simulink model "net_model_2_nodes"  (R2024a)
settings: Solver=VariableStepAuto  StartTime=0.0  StopTime=100  RelTol=1e-3
values from neighbouring files (symbols this model uses):
  A = [A11, A12 ... (first row only)    [main.m]
  B = blkdiag(B, B)    [main.m]
  C = blkdiag(C, C)    [main.m]
  L = [0, 1 ... (first row only)    [main.m]
  node_1_0 = [0; 0]    [main.m]
  node_2_0 = [0; 0]    [main.m]
settings Model: Creator=antoniostavarache  LastModifiedBy=antoniostavarache

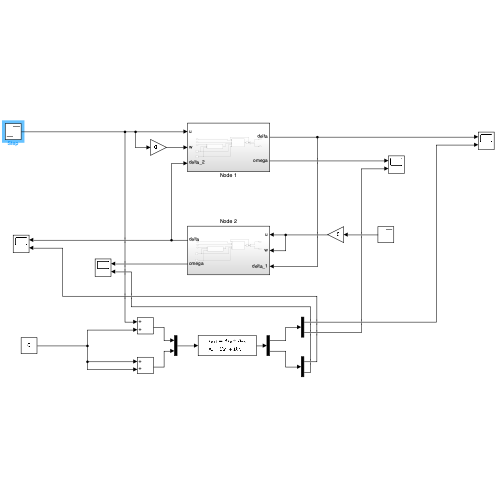
[thumbnail: Simulink's stored preview of the top-level diagram]
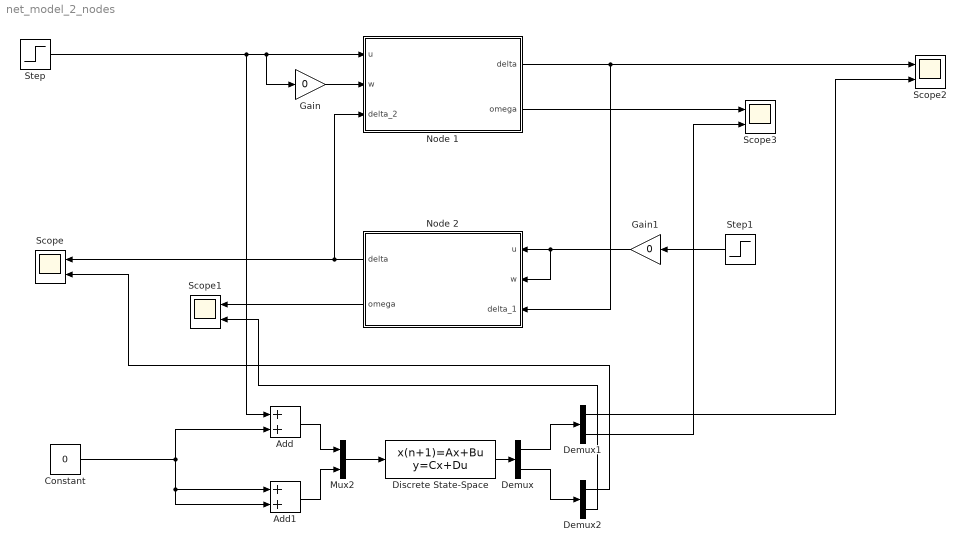
== system net_model_2_nodes ==
  Add : Sum
  Add1 : Sum
  Constant : Constant  Value=0
  Demux : Demux  Outputs=2
  Demux1 : Demux  Outputs=2
  Demux2 : Demux  Outputs=2
  Discrete State-Space : DiscreteStateSpace  A=A  B=B  C=C  D=zeros(4, 2)
  Gain : Gain  Gain=0
  Gain1 : Gain  Gain=0
  Mux2 : Mux  Inputs=2
  Node 1 : Subsystem
  Node 2 : Subsystem
  Scope{,1..3} (4 alike) : Scope  NumInputPorts=2
  Step : Step  SampleTime=0
  Step1 : Step  SampleTime=0
  wires:
  Node 1/1(delta) -> Scope2/1, Node 2/3(delta_1)
  Node 2/1(delta) -> Node 1/3(delta_2), Scope/1
  Node 2/2(omega) -> Scope1/1
  Node 1/2(omega) -> Scope3/1
  Step/1 -> Add/1, Node 1/1(u), Gain/1
  Gain/1 -> Node 1/2(w)
  Step1/1 -> Gain1/1
  Gain1/1 -> Node 2/2(w), Node 2/1(u)
  Constant/1 -> Add1/2, Add1/1, Add/2
  Add/1 -> Mux2/1
  Add1/1 -> Mux2/2
  Demux/1 -> Demux1/1
  Demux/2 -> Demux2/1
  Demux1/1 -> Scope2/2
  Demux1/2 -> Scope3/2
  Demux2/1 -> Scope/2
  Demux2/2 -> Scope1/2
  Mux2/1 -> Discrete State-Space/1
  Discrete State-Space/1 -> Demux/1

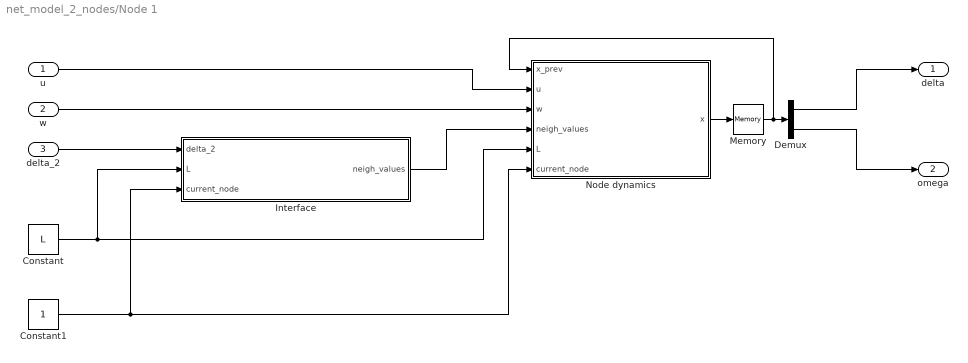
== system net_model_2_nodes/Node 1 ==
  u : Inport
  w : Inport  Port=2
  delta_2 : Inport  Port=3
  Constant : Constant  Value=L
  Constant1 : Constant
  Demux : Demux  Outputs=2
  Interface : MATLAB Function  TreatAsAtomicUnit=on
  Memory : Memory  InitialCondition=node_1_0
  Node dynamics : MATLAB Function  TreatAsAtomicUnit=on
  delta : Outport
  omega : Outport  Port=2
  wires:
  Node dynamics/1(x) -> Memory/1
  Interface/1(neigh_values) -> Node dynamics/4(neigh_values)
  Constant/1 -> Node dynamics/5(L), Interface/2(L)
  Constant1/1 -> Node dynamics/6(current_node), Interface/3(current_node)
  u/1 -> Node dynamics/2(u)
  w/1 -> Node dynamics/3(w)
  Demux/1 -> delta/1
  Demux/2 -> omega/1
  delta_2/1 -> Interface/1(delta_2)
  Memory/1 -> Node dynamics/1(x_prev), Demux/1

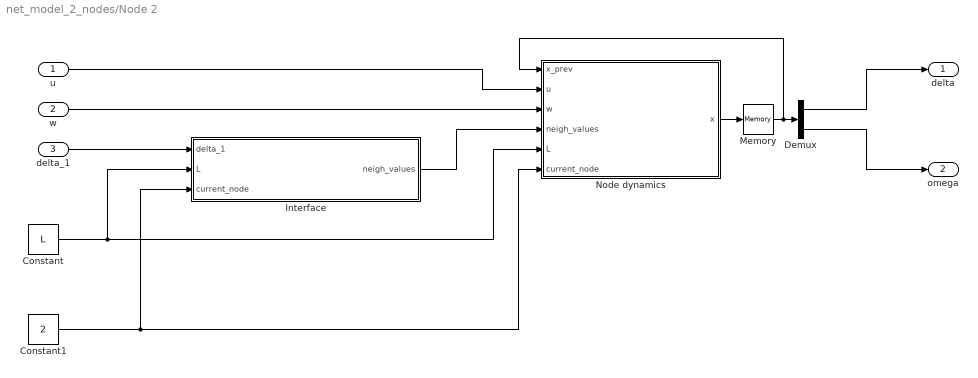
== system net_model_2_nodes/Node 2 ==
  u : Inport
  w : Inport  Port=2
  delta_1 : Inport  Port=3
  Constant : Constant  Value=L
  Constant1 : Constant  Value=2
  Demux : Demux  Outputs=2
  Interface : MATLAB Function  TreatAsAtomicUnit=on
  Memory : Memory  InitialCondition=node_2_0
  Node dynamics : MATLAB Function  TreatAsAtomicUnit=on
  delta : Outport
  omega : Outport  Port=2
  wires:
  Node dynamics/1(x) -> Memory/1
  Interface/1(neigh_values) -> Node dynamics/4(neigh_values)
  Constant/1 -> Node dynamics/5(L), Interface/2(L)
  Constant1/1 -> Node dynamics/6(current_node), Interface/3(current_node)
  u/1 -> Node dynamics/2(u)
  w/1 -> Node dynamics/3(w)
  Demux/1 -> delta/1
  Demux/2 -> omega/1
  delta_1/1 -> Interface/1(delta_1)
  Memory/1 -> Node dynamics/1(x_prev), Demux/1

== matlab function net_model_2_nodes/Node 1/Interface ==
  data: delta_2 input; neigh_values output; L input; current_node input
function neigh_values = fcn(delta_2, L, current_node)
    
    % curr_node = 1;

    % l_mat = [0 0.6511 0.7915 0 0.7513;
    %     0.6511 0 0 0.8433 0.6318;
    %     0.7915 0 0 0.8259 0.8620;
    %     0 0.8433 0.8259 0 0.8367;
    %     0.7513 0.6318 0.8620 0.8367 0];

    l_mat = [0 0.6511;
        0.6511 0];

    neigh_values = L(current_node, 2) * l_mat(current_node, 2) * delta_2;

end

== matlab function net_model_2_nodes/Node 1/Node dynamics ==
  data: x_prev input; u input; x output; w input; neigh_values input; L input; current_node input
function x = fcn(x_prev, u, w, neigh_values, L, current_node)
    
    % current_node = 1;

%%

    hi = [0.3244
        1.5886];

    di = [0.5650;
        0.7844];
    
    l_mat = [0 0.6511;
        0.6511 0];

    dt = 0.2;
%%

    a21 = -hi(current_node) * dt * L(current_node, :) * l_mat(current_node, :)';
    a22 = 1 - hi(current_node) * di(current_node) * dt;

    A = [1, dt;
        a21, a22];

    x = A * x_prev + [0 1]' * (u + w + hi(current_node) * dt * neigh_values);
    
end

== matlab function net_model_2_nodes/Node 2/Interface ==
  data: delta_1 input; neigh_values output; L input; current_node input
function neigh_values = fcn(delta_1, L, current_node)
    
    % curr_node = 1;

    % l_mat = [0 0.6511 0.7915 0 0.7513;
    %     0.6511 0 0 0.8433 0.6318;
    %     0.7915 0 0 0.8259 0.8620;
    %     0 0.8433 0.8259 0 0.8367;
    %     0.7513 0.6318 0.8620 0.8367 0];

    l_mat = [0 0.6511;
        0.6511 0];

    neigh_values = L(current_node, 1) * l_mat(current_node, 1) * delta_1;

end

== matlab function net_model_2_nodes/Node 2/Node dynamics ==
  data: x_prev input; u input; x output; w input; neigh_values input; L input; current_node input
function x = fcn(x_prev, u, w, neigh_values, L, current_node)
    
    % current_node = 1;

%%

    hi = [0.3244
        1.5886];

    di = [0.5650;
        0.7844];
    
    l_mat = [0 0.6511;
        0.6511 0];

    dt = 0.2;
    
%%

    a21 = -hi(current_node) * dt * L(current_node, :) * l_mat(current_node, :)';
    a22 = 1 - hi(current_node) * di(current_node) * dt;

    A = [1, dt;
        a21, a22];

    x = A * x_prev + [0 1]' * (u + w + hi(current_node) * dt * neigh_values);
    
end
